simulink model "CompleteAttDetSim"  (R2018b)
settings: Solver=FixedStepAuto  StartTime=0.0  StopTime=24*3600  FixedStep=10  RelTol=1e-3  EnableMultiTasking=on
PreLoadFcn:
  | InitialiseJ2
values from neighbouring files (symbols this model uses):
  AngMomentum = (grav_parameter*rp*(1 + eccentricity))^0.5    [InitialiseJ2.m]
  Arg_periapsis = D3(1,6)    [InitialiseJ2.m]
  earthRadius = 6378.137    [InitialiseJ2.m]
  eccentricity = D3(1,5)/1e7    [InitialiseJ2.m]
  grav_parameter = 398600.4415    [InitialiseJ2.m]
  inclination = D3(1,3)    [InitialiseJ2.m]
  J2 = 0.0010836    [InitialiseJ2.m]
  period = 2*pi*sqrt(sm_axis^3/grav_parameter)    [InitialiseJ2.m]
  RAAN = D3(1,4)    [InitialiseJ2.m]
  sm_axis = (grav_parameter/(avg_motion*2*pi/(24*3600))^2)^(1/3)    [InitialiseJ2.m]
  t0 = avg_anomaly/(2*pi)*period    [InitialiseJ2.m]
undefined symbols (not defined in the file or in its folder): Earth, WGS84
libraries: vrlib x11, sharedtransform x7, simulink x6, aerolibutil x4, aerolibtransform2 x1
(part 2 of 2)

== matlab function CompleteAttDetSim/IGRF/Magnetic Field in Local Spherical Coordinates ==
  data: lat input; Brad output; long input; Geodectic_rad input; date input; Btheat output; Bphi output; geoclatitude output; simtime input

function [Brad,Btheat,Bphi,geoclatitude] = Magfield_Spherical(lat,long,Geodectic_rad,date, simtime)
%Magnetic field in Spherical Coordinates

if (lat>-0.00000001 && lat<0.00000001)
    lat=0.00000001;
    
elseif(lat<180.00000001 && lat>179.99999999)
    lat=179.99999999;
end

costheta = cos((90 - lat)*pi/180);
sintheta = sin((90 - lat)*pi/180);

 ra = 6378.137; f = 1/298.257223563; b = ra*(1 - f);
    rho = hypot(ra*sintheta, b*costheta);
    r = sqrt( Geodectic_rad.^2 + 2*Geodectic_rad.*rho + ...
        (ra^4*sintheta.^2 + b^4*costheta.^2) ./ rho.^2 );
    cd = (Geodectic_rad + rho) ./ r;
    sd = (ra^2 - b^2) ./ rho .* costheta.*sintheta./r;
    oldcos = costheta;
    costheta = costheta.*cd - sintheta.*sd;
    sintheta = sintheta.*cd + oldcos.*sd;
    geoclatitude=90-acos(costheta)*180/pi;
 phi = long*pi/180;

setdate=[2015 1 1 0 0 0];
givenjd=findjd(date)+simtime/86400;
setjd=findjd(setdate);
days=givenjd-setjd;

a=6371.2; 

 gm=[0;1;0;1;2;0;1;2;3;0;1;2;3;4;0;1;2;3;4;5;0;1;2;3;4;5;6;0;1;2;3;4;5;6;7;0;1;2;3;4;5;6;7;8;0;1;2;3;4;5;6;7;8;9;0;1;2;3;4;5;6;7;8;9;10;0;1;2;3;4;5;6;7;8;9;10;11;0;1;2;3;4;5;6;7;8;9;10;11;12;0;1;2;3;4;5;6;7;8;9;10;11;12;13];
 gn=[1;1;2;2;2;3;3;3;3;4;4;4;4;4;5;5;5;5;5;5;6;6;6;6;6;6;6;7;7;7;7;7;7;7;7;8;8;8;8;8;8;8;8;8;9;9;9;9;9;9;9;9;9;9;10;10;10;10;10;10;10;10;10;10;10;11;11;11;11;11;11;11;11;11;11;11;11;12;12;12;12;12;12;12;12;12;12;12;12;12;13;13;13;13;13;13;13;13;13;13;13;13;13;13];
 gsvi=[10.3000000000000;18.1000000000000;-13.0500000000000;-5.71580000000000;1.81870000000000;8.50000000000000;-16.8400000000000;-1.35550000000000;-7.98480000000000;-3.06250000000000;1.10680000000000;-35.6090000000000;8.57580000000000;-3.17990000000000;-1.57500000000000;5.08330000000000;-9.99080000000000;-0.470620000000000;3.10590000000000;2.73610000000000;-4.33120000000000;-1.89030000000000;-10.4610000000000;20.9220000000000;-6.54820000000000;0.698040000000000;1.07470000000000;8.04370000000000;-7.09390000000000;-14.4800000000000;26.6220000000000;1.23490000000000;-3.70470000000000;-1.93750000000000;0.129450000000000;10.0550000000000;0;-33.6490000000000;20.7100000000000;-5.34720000000000;5.93220000000000;0.686520000000000;-1.00270000000000;0.188010000000000;0;0;0;0;0;0;0;0;0;0;0;0;0;0;0;0;0;0;0;0;0;0;0;0;0;0;0;0;0;0;0;0;0;0;0;0;0;0;0;0;0;0;0;0;0;0;0;0;0;0;0;0;0;0;0;0;0;0;0;0];
 gvali=[-29442;-1501;-3667.60000000000;5218.50000000000;1452.10000000000;3376.80000000000;-7202.40000000000;2373.40000000000;460.110000000000;3970.80000000000;4503;471.140000000000;-700.490000000000;52.0620000000000;-1831.70000000000;3661;1478.60000000000;-663.110000000000;-349.420000000000;2.87640000000000;1010.60000000000;1279.70000000000;1086.40000000000;-1294.20000000000;-157.700000000000;30.7140000000000;-47.6230000000000;2187.90000000000;-2699.20000000000;-196.930000000000;1060.80000000000;185.230000000000;58.0400000000000;-6.78110000000000;4.40140000000000;1216.60000000000;589.880000000000;-947.790000000000;-132.540000000000;-550.770000000000;198.730000000000;80.3230000000000;-39.8590000000000;-1.25340000000000;512.790000000000;1121.20000000000;336.820000000000;-273.840000000000;39.4630000000000;-448.090000000000;-1.73980000000000;65.5420000000000;-23.5140000000000;-6.39500000000000;-342.810000000000;-1532.70000000000;21.0690000000000;82.6400000000000;-58.4350000000000;133.050000000000;-28.9240000000000;42.0910000000000;19.6380000000000;-4.77860000000000;-2.13710000000000;1067.80000000000;-699.580000000000;-940.810000000000;655.940000000000;-191.610000000000;95.0540000000000;-65.8820000000000;9.92090000000000;38.6920000000000;-1.76300000000000;1.08810000000000;2.02990000000000;-1254.40000000000;-179.410000000000;318.050000000000;779.060000000000;-389.530000000000;300.620000000000;20.8300000000000;58.5270000000000;-17.5580000000000;-10.2170000000000;1.88650000000000;-2.50330000000000;0;0;-1557.20000000000;619.010000000000;641.570000000000;-492.060000000000;695.880000000000;-90.3090000000000;213.710000000000;-14.2790000000000;20.4220000000000;2.83880000000000;5.01840000000000;-1.13550000000000;-0.167020000000000];
     
 hm=[0;1;0;1;2;0;1;2;3;0;1;2;3;4;0;1;2;3;4;5;0;1;2;3;4;5;6;0;1;2;3;4;5;6;7;0;1;2;3;4;5;6;7;8;0;1;2;3;4;5;6;7;8;9;0;1;2;3;4;5;6;7;8;9;10;0;1;2;3;4;5;6;7;8;9;10;11;0;1;2;3;4;5;6;7;8;9;10;11;12;0;1;2;3;4;5;6;7;8;9;10;11;12;13];
 hn=[1;1;2;2;2;3;3;3;3;4;4;4;4;4;5;5;5;5;5;5;6;6;6;6;6;6;6;7;7;7;7;7;7;7;7;8;8;8;8;8;8;8;8;8;9;9;9;9;9;9;9;9;9;9;10;10;10;10;10;10;10;10;10;10;10;11;11;11;11;11;11;11;11;11;11;11;11;12;12;12;12;12;12;12;12;12;12;12;12;12;13;13;13;13;13;13;13;13;13;13;13;13;13;13];
 hsvi=[0;-26.6000000000000;0;-47.4580000000000;-12.2110000000000;0;25.1070000000000;-0.774600000000000;1.42300000000000;0;-7.19420000000000;20.7400000000000;6.06580000000000;-3.84550000000000;0;6.09990000000000;13.0650000000000;-5.64750000000000;7.54300000000000;0;0;0;-31.3830000000000;-6.97400000000000;1.09140000000000;2.09410000000000;0.671690000000000;0;28.3760000000000;11.5840000000000;-4.09570000000000;-3.70470000000000;-3.70470000000000;0.242180000000000;-0.129450000000000;0;-20.1090000000000;16.8250000000000;4.14200000000000;13.3680000000000;-2.96610000000000;-2.05960000000000;0.752050000000000;0;0;0;0;0;0;0;0;0;0;0;0;0;0;0;0;0;0;0;0;0;0;0;0;0;0;0;0;0;0;0;0;0;0;0;0;0;0;0;0;0;0;0;0;0;0;0;0;0;0;0;0;0;0;0;0;0;0;0;0;0];
 hvali=[0;4797.10000000000;0;-4928.70000000000;-555.900000000000;0;-353.030000000000;474.250000000000;-425.640000000000;0;1567.80000000000;-738.410000000000;378.380000000000;-243.670000000000;0;480.880000000000;1514;-561.450000000000;35.4960000000000;70.2960000000000;0;-393.180000000000;496.150000000000;586.810000000000;-363.970000000000;16.9860000000000;42.0480000000000;0;-1918.90000000000;-564.740000000000;116.730000000000;301.310000000000;20.9930000000000;-66.3580000000000;-1.42400000000000;0;677.020000000000;-1026.30000000000;550.880000000000;-390.350000000000;240.260000000000;39.1320000000000;-22.8120000000000;1.31610000000000;0;-2751.90000000000;1173.40000000000;979.200000000000;-383.360000000000;-232.470000000000;135.700000000000;7.53350000000000;-10.3360000000000;5.11600000000000;0;778.520000000000;-84.2770000000000;760.290000000000;514.230000000000;-583.930000000000;-24.7920000000000;-84.1810000000000;-22.9110000000000;-3.18570000000000;-5.16460000000000;0;-46.6390000000000;818.100000000000;-229.580000000000;-263.470000000000;126.740000000000;-18.8240000000000;-109.130000000000;-31.8640000000000;-22.0370000000000;-5.44070000000000;-1.39200000000000;0;-986.730000000000;318.050000000000;1233.50000000000;-1071.20000000000;100.210000000000;145.810000000000;-11.7050000000000;17.5580000000000;5.10870000000000;-8.48920000000000;-0.278150000000000;0.397440000000000;0;-1557.20000000000;619.010000000000;2053;-492.060000000000;-835.050000000000;-45.1550000000000;106.860000000000;-14.2790000000000;27.2290000000000;14.1940000000000;-3.01100000000000;-1.13550000000000;-0.445390000000000];


N=max(gn);
g=zeros(N,N+1);
Geodectic_rad=zeros(N,N+1);
for x=1:length(gn)
    g(gn(x),gm(x)+1) = gvali(x) + gsvi(x)*days/365;
    Geodectic_rad(hn(x),hm(x)+1) = hvali(x) + hsvi(x)*days/365;
end

Brad=0; Btheat=0; Bphi=0; P20=0; dP20=0;
P11=1; P10=P11;
dP11=0; dP10=dP11;
for m=0:N
    for n=1:N
        if m<=n
            % Calculate Legendre polynomials and derivatives recursively
            if n==m
                P2 = sintheta*P11;
                dP2 = sintheta*dP11 + costheta*P11;
                P11=P2; P10=P11; P20=0;
                dP11=dP2; dP10=dP11; dP20=0;
            elseif n==1
                  P2 = costheta*P10;
                  dP2 = costheta*dP10 - sintheta*P10;
                  P20=P10; P10=P2;
                  dP20=dP10; dP10=dP2;
            else
                K = ((n-1)^2-m^2)/((2*n-1)*(2*n-3));
                P2 = costheta*P10 - K*P20;
                dP2 = costheta*dP10 - sintheta*P10 - K*dP20;
                P20=P10; P10=P2;
                dP20=dP10; dP10=dP2;
            end
            
            % Calculate Br, Bt, and Bp
            Brad = Brad + (a/r)^(n+2)*(n+1)*...
                ((g(n,m+1)*cos(m*phi) + Geodectic_rad(n,m+1)*sin(m*phi))*P2);
            Btheat = Btheat + (a/r)^(n+2)*...
                ((g(n,m+1)*cos(m*phi) + Geodectic_rad(n,m+1)*sin(m*phi))*dP2);
            Bphi = Bphi + (a/r)^(n+2)*...
                (m*(-g(n,m+1)*sin(m*phi) + Geodectic_rad(n,m+1)*cos(m*phi))* P2);
        end
    end
end
Btheat =-Btheat;
Bphi= -(Bphi/(sintheta));
end
function jd=findjd(datevec)
yr=datevec(1); mon=datevec(2); day=datevec(3); hr=datevec(4); min=datevec(5); sec=datevec(6);
        jd = 367.0 * yr  ...
             - floor( (7 * (yr + floor( (mon + 9) / 12.0) ) ) * 0.25 )   ...
             + floor( 275 * mon / 9.0 ) ...
             + day + 1721013.5  ...
             + ( (sec/60.0 + min ) / 60.0 + hr ) / 24.0;
end

    function c=hypota(a,b)
        c = sqrt(abs(a).^2 + abs(b).^2)
    end

== matlab function CompleteAttDetSim/Sun Sensor/Random Quat Error ==
  data: quat output
function quat = errorquatgen()
%generate quaternion for rotation of given angle (rad) around random axis
%computing first term of quaternion
angle=normrnd(0,0.0029);
q0=cos(angle/2);
%random axis
a=rand;
b=rand;
c=rand;
axis=[a b c];
%normalise the random axis
n=norm(axis);
a=a/n;
b=b/n;
c=c/n;
%computing quaternoin
q1=a*sin(angle/2);
q2=b*sin(angle/2);
q3=c*sin(angle/2);
quat=[q0 q1 q2 q3];
end

== matlab function CompleteAttDetSim/ Sun Position/Fraction Of Day ==
  data: uthr input; fracjd output; utmin input; utsec input
function fracjd=fracjday(uthr, utmin, utsec)
fracjd=uthr / 24 + utmin / 1440 + utsec / 86400;

== matlab function CompleteAttDetSim/ Sun Position/Julian Date ==
  data: month input; wholejd output; day input; year input
function wholejd = julian (month, day, year)
wholejd=0;
y = year;
m = month;
b = 0;
c = 0;

if (m <= 2)
   y = y - 1;
   m = m + 12;
end

if (y < 0)
   c = -.75;
end

% check for valid calendar date
if (year < 1582)
   % null
elseif (year > 1582)
   a = fix(y / 100);
   b = 2 - a + floor(a / 4);
elseif (month < 10)
   % null
elseif (month > 10)
   a = fix(y / 100);
   b = 2 - a + floor(a / 4);
elseif (day <= 4)
   % null
elseif (day > 14)
   a = fix(y / 100);
   b = 2 - a + floor(a / 4);  
   fprintf('\n\n  this is an invalid calendar date!!\n');
   return;
end

jd = fix(365.25 * y + c) + fix(30.6001 * (m + 1));
wholejd = jd + day + b + 1720994.5;

== matlab function CompleteAttDetSim/ Sun Position/Sun Position ECI ==
  data: jdate input; rsun output
function rsun  = sun1 (jdate)
atr = pi / 648000;
rsun = zeros(3, 1);

% time arguments
djd = jdate - 2451545;
t = (djd / 36525) + 1;

% fundamental arguments (radians)
gs =2.0*pi*((0.993126+0.0027377785*djd)-fix(0.993126+0.0027377785*djd));
lm = 2.0*pi*((0.606434+0.03660110129*djd)-fix(0.606434+0.03660110129*djd));
ls = 2.0*pi*((0.606434+0.03660110129*djd)-fix(0.606434+0.03660110129*djd));
g2 = 2.0*pi*((0.606434+0.03660110129*djd)-fix(0.606434+0.03660110129*djd));
g4 = 2.0*pi*((0.606434+0.03660110129*djd)-fix(0.606434+0.03660110129*djd));
g5 = 2.0*pi*((0.606434+0.03660110129*djd)-fix(0.606434+0.03660110129*djd));
rm = 2.0*pi*((0.606434+0.03660110129*djd)-fix(0.606434+0.03660110129*djd));

% geocentric, ecliptic longitude of the sun (radians)
plon = 6910*sin(gs)+72*sin(2*gs)-17*t*sin(gs);
plon = plon-7*cos(gs-g5)+6*sin(lm-ls)+5*sin(4*gs-8*g4+3*g5);
plon = plon-5*cos(2*(gs-g2))-4*(sin(gs-g2)-cos(4*gs-8*g4+3*g5));
plon = plon+3*(sin(2*(gs-g2))-sin(g5)-sin(2*(gs-g5)));
plon = ls+atr*(plon-17*sin(rm));

% geocentric distance of the sun (kilometers)
rsm = 149597870.691*(1.00014-0.01675*cos(gs)-0.00014*cos(2*gs));

% obliquity of the ecliptic (radians)
obliq = atr*(84428-47*t+9*cos(rm));

% geocentric, equatorial right ascension and declination (radians)
a = sin(plon)*cos(obliq);
b = cos(plon);

epsilon = 0.0000000001;
pidiv2 = 0.5 * pi;
dontenterflag=0;
c=0;
if (abs(a) < epsilon)
    rascy = (1 - sign(b)) * pidiv2;
    dontenterflag=1;
else
    c = (2 - sign(a)) * pidiv2;
end
if ((abs(b) < epsilon)&&dontenterflag~=1)
    rascy = c;
else
    rascy = c + sign(a) * sign(b) * (abs(atan(a / b)) - pidiv2);
end
rasc = rascy;
decl = asin(sin(obliq) * sin(plon));

% geocentric position vector of the sun (kilometers)
rsun(1) = rsm * cos(rasc) * cos(decl);
rsun(2) = rsm * sin(rasc) * cos(decl);
rsun(3) = rsm * sin(decl);

== matlab function CompleteAttDetSim/Model Attitude Martix/Rotate about x1 ==
  data: u input; y output
function y = fcn(u)
y =rotx(u);

== matlab function CompleteAttDetSim/Attitude Propagator/TRIAD ==
  data: ref1 input; Attitude_Matrix output; ref2 input; vec1 input; vec2 input
function Attitude_Matrix=Triad(ref1,ref2,vec1,vec2)

%To avoid error of both vectors having same cross product
if ref1==ref2
    ref2(1)=ref2(1)+ 0.00000000000000001;
end
if vec1==vec2
    vec2(1)=vec2(1)+ 0.00000000000000001;
end

%Calculate body tirad
triad1body=vec1./norm(vec1);
triad2body=cross(triad1body,vec2)./norm(cross(triad1body,vec2));
triad3body=cross(triad1body,triad2body)./norm(cross(triad1body,triad2body));

%Calculate reference tirad
triad1ref=ref1./norm(ref1);
triad2ref=cross(triad1ref,ref2)./norm(cross(triad1ref,ref2));
triad3ref=cross(triad1ref,triad2ref)./norm(cross(triad1ref,triad2ref));

%Calculate attituce matrix
Attitude_Matrix= triad1body*(triad1ref.') + triad2body*(triad2ref.') + triad3body*(triad3ref.');

== matlab function CompleteAttDetSim/Optimised Triad/MATLAB Function ==
  data: A1 input; Attitude_Matrix output; A2 input
function Attitude_Matrix=Optimised_Triad(A1,A2)
sigma1=0.01; %noise
sigma2=0.1;
LinearEstimator=((sigma2)^2/((sigma1)^2+(sigma2)^2))...
    *A1+((sigma1)^2/((sigma1)^2+(sigma2)^2))*A2;
%Orthogonalise
Attitude_Matrix=0.5*(LinearEstimator+(inv(LinearEstimator).'));

== matlab function CompleteAttDetSim/Optimised Triad/Triad Using 1 as anchor vector ==
  data: ref1 input; ref2 input; vec1 input; vec2 input; A1 output
function A1=Triad(ref1,ref2,vec1,vec2)
%This function generates an attitude matrix two reference and two measured
%vectors.

%Calculate body tirad
triad1body=vec1./norm(vec1);
triad2body=cross(triad1body,vec2)./norm(cross(triad1body,vec2));
triad3body=cross(triad1body,triad2body)./norm(cross(triad1body,triad2body));

%Calculate reference tirad
triad1rot=ref1./norm(ref1);
triad2rot=cross(triad1rot,ref2)./norm(cross(triad1rot,ref2));
triad3rot=cross(triad1rot,triad2rot)./norm(cross(triad1rot,triad2rot));

%Calculate attituce matrix
A1= triad1body*(triad1rot.') + triad2body*(triad2rot.') + triad3body*(triad3rot.');

== matlab function CompleteAttDetSim/Optimised Triad/Triad Using 2 as anchor vector ==
  data: ref1 input; A2 output; ref2 input; vec1 input; vec2 input
function A2=Triad(ref1,ref2,vec1,vec2)

%Calculate body tirad
triad1body=vec1./norm(vec1);
triad2body=cross(triad1body,vec2)./norm(cross(triad1body,vec2));
triad3body=cross(triad1body,triad2body)./norm(cross(triad1body,triad2body));

%Calculate reference tirad
triad1rot=ref1./norm(ref1);
triad2rot=cross(triad1rot,ref2)./norm(cross(triad1rot,ref2));
triad3rot=cross(triad1rot,triad2rot)./norm(cross(triad1rot,triad2rot));

%Calculate attituce matrix
A2= triad1body*(triad1rot.') + triad2body*(triad2rot.') + triad3body*(triad3rot.');

== matlab function CompleteAttDetSim/ Magnetometer/Magnetometer Error/Add Error ==
  data: y output
function y = NoiseGenerator()
RSS_err=0.12*1/100; 
FullScale=0.8;  
y=randn(3,1)*RSS_err*FullScale;
end

== matlab function CompleteAttDetSim/Control Law ==
  data: magField input; m output; angvel input; angvel output
function [m, angvel]  = bdot(magField, angvel)
%reads in magnetic field vector in body coordinates,and angular velocity

% % B-dot Control 
detb=sqrt(dot((magField),(magField)));    
m=((-1)/detb)*cross(magField,angvel); %actuation level

torque=cross(m,magField);
inertia=[0.00602377522,0.00000294634,0.00000423169;0.00000294634,0.00130455071,0.00001311622;0.00000294634,0.00001311622,0.00601351576]';
angacc=torque'/inertia;
angvel=angvel+(angacc*0.1)';%calculates the new angular velocity


% % magField=magField(x,:);
% % angvel=angvel(x,:);
% %     
% % % B-dot Control 
% % detb=sqrt(dot((magField),(magField)));    
% % m=((-1)/detb)*cross(magField,angvel); %actuation level
% % 
% % 
% % torque=cross(m,magField);
% % inertia=[0.00602377522,0.00000294634,0.00000423169;0.00000294634,0.00130455071,0.00001311622;0.00000294634,0.00001311622,0.00601351576]';
% % angacc=torque'/inertia;
% % angvel=angvel+(angacc*0.1)';%calculates the new angular velocity
     
 end
